simulink model "L1_Control_with_fallback"  (Simulink 7.9)
settings: Solver=ode45  StartTime=0.0  StopTime=300  FixedStep=0.02  MaxStep=0.1  RelTol=1e-3
libraries: simulink x7
settings Model: Creator=prisebor  LastModifiedBy=user
settings SolverCC: ZeroCrossAlgorithm=Adaptive  AutoInsertRateTranBlk=on
settings GRTTargetCC: CombineOutputUpdateFcns=off  GRTInterface=on

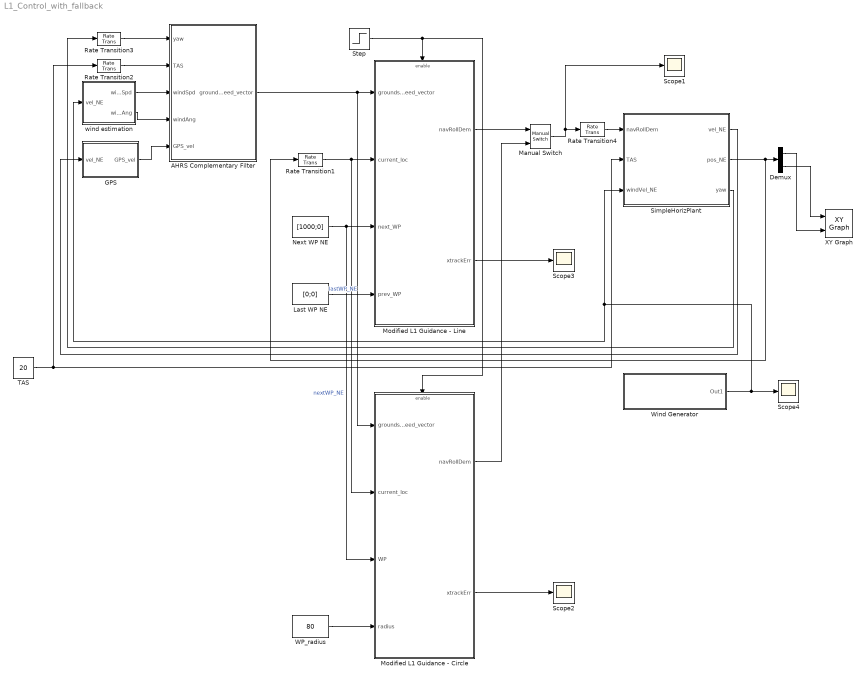
== system L1_Control_with_fallback ==
  AHRS Complementary Filter : Subsystem  TreatAsAtomicUnit=on  SystemSampleTime=0.1
  Demux : Demux  Outputs=2
  GPS : Subsystem  SystemSampleTime=0.2
  Last WP NE : Constant  Value=[0;0]  SampleTime=0.1
  Manual Switch : simulink/Signal Routing/Manual Switch  sw=1  action=0  varsize=off
  Modified L1 Guidance - Circle : Subsystem  TreatAsAtomicUnit=on  SystemSampleTime=0.1  mask{period=20, dampingRatio=0.71, loitDirn=-1}
      mask prompts: period "Tracking Loop Period (sec) - set to 15 times total loop delay"; dampingRatio "Tracking Loop Theoretical Damping Ratio"; loitDirn "Loiter Direction [1 , -1] - 1 for RH, -1 for LH"
  Modified L1 Guidance - Line : Subsystem  TreatAsAtomicUnit=on  SystemSampleTime=0.1  mask{period=20, dampingRatio=0.71, fallbackEnable=1}
      mask prompts: period "Tracking Loop Period (sec) - set to 15 times total loop delay"; dampingRatio "Tracking Loop Theoretical Damping Ratio"; fallbackEnable "Enables fallback mode [1=enabled, 0=disabled]"
  Next WP NE : Constant  Value=[1000;0]  SampleTime=0.1
  Rate Transition1 : RateTransition  OutPortSampleTime=0.1
  Rate Transition2 : RateTransition  OutPortSampleTime=0.1
  Rate Transition3 : RateTransition  OutPortSampleTime=0.1
  Rate Transition4 : RateTransition  OutPortSampleTime=0
  Scope{1..4} (4 alike) : Scope
      Scope2 settings: SaveName=ScopeData2
      Scope4 settings: YMin=-15  SaveName=ScopeData3
  SimpleHorizPlant : Subsystem
  Step : Step  SampleTime=0
  TAS : Constant  Value=20  SampleTime=0
  WP_radius : Constant  Value=80  SampleTime=0.1
  Wind Generator : Subsystem
  XY Graph : simulink/Sinks/XY Graph  xmin=-1000  xmax=1000  ymin=-1000  ymax=1000  st=-1
  wind estimation : Subsystem  SystemSampleTime=0.2
  wires:
  Next WP NE/1 -> Modified L1 Guidance - Circle/3(WP), Modified L1 Guidance - Line/3(next_WP)  "nextWP_NE"
  Last WP NE/1 -> Modified L1 Guidance - Line/4(prev_WP)  "lastWP_NE"
  SimpleHorizPlant/2(pos_NE) -> Rate Transition1/1, Demux/1
  TAS/1 -> SimpleHorizPlant/2(TAS), Rate Transition2/1
  SimpleHorizPlant/3(yaw) -> Rate Transition3/1
  Wind Generator/1(Out1) -> SimpleHorizPlant/3(windVel_NE), wind estimation/1(vel_NE), Scope4/1
  Modified L1 Guidance - Line/1(navRollDem) -> Manual Switch/1
  Rate Transition1/1 -> Modified L1 Guidance - Circle/2(current_loc), Modified L1 Guidance - Line/2(current_loc)
  Rate Transition4/1 -> SimpleHorizPlant/1(navRollDem)
  wind estimation/1(windSpd) -> AHRS Complementary Filter/3(windSpd)
  wind estimation/2(windAng) -> AHRS Complementary Filter/4(windAng)
  Rate Transition3/1 -> AHRS Complementary Filter/1(yaw)
  Rate Transition2/1 -> AHRS Complementary Filter/2(TAS)
  SimpleHorizPlant/1(vel_NE) -> GPS/1(vel_NE)
  GPS/1(GPS_vel) -> AHRS Complementary Filter/5(GPS_vel)
  AHRS Complementary Filter/1(groundspeed_vector) -> Modified L1 Guidance - Circle/1(groundspeed_vector), Modified L1 Guidance - Line/1(groundspeed_vector)
  WP_radius/1 -> Modified L1 Guidance - Circle/4(radius)
  Step/1 -> Modified L1 Guidance - Circle/Enable, Modified L1 Guidance - Line/Enable
  Demux/1 -> XY Graph/2
  Demux/2 -> XY Graph/1
  Manual Switch/1 -> Scope1/1, Rate Transition4/1
  Modified L1 Guidance - Circle/1(navRollDem) -> Manual Switch/2
  Modified L1 Guidance - Circle/2(xtrackErr) -> Scope2/1
  Modified L1 Guidance - Line/2(xtrackErr) -> Scope3/1

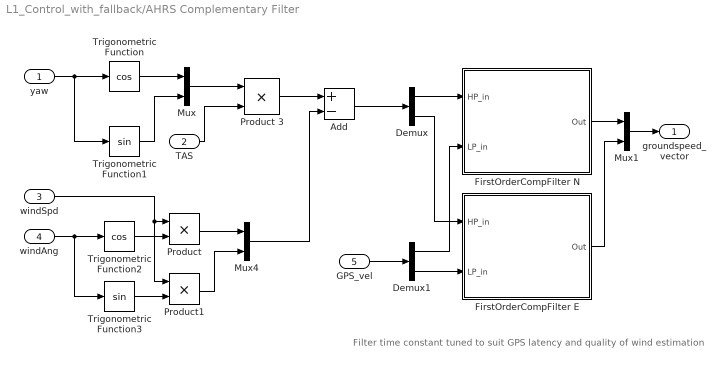
== system L1_Control_with_fallback/AHRS Complementary Filter ==
  note: Filter time constant tuned to suit GPS latency and quality of wind estimation
  yaw : Inport
  TAS : Inport  Port=2
  windSpd : Inport  Port=3
  windAng : Inport  Port=4
  GPS_vel : Inport  Port=5
  Add : Sum  Inputs=+-
  Demux : Demux  Outputs=2
  Demux1 : Demux  Outputs=2
  FirstOrderCompFilter E : Subsystem  mask{beta=0.1}
      mask prompts: beta "Beta=dt/Tau, Tau = filter time constant (sec), dt = filter time step (sec)"
  FirstOrderCompFilter N : Subsystem  mask{beta=0.1}
      mask prompts: beta "Beta=dt/Tau, Tau = filter time constant (sec), dt = filter time step (sec)"
  Mux : Mux  Inputs=2
  Mux1 : Mux  Inputs=2
  Mux4 : Mux  Inputs=2
  Product : Product  RndMeth=Zero
  Product 3 : Product  RndMeth=Zero
  Product1 : Product  RndMeth=Zero
  Trigonometric Function : Trigonometry  Operator=cos
  Trigonometric Function1 : Trigonometry
  Trigonometric Function2 : Trigonometry  Operator=cos
  Trigonometric Function3 : Trigonometry
  groundspeed_vector : Outport
  wires:
  yaw/1 -> Trigonometric Function/1, Trigonometric Function1/1
  Trigonometric Function/1 -> Mux/1
  Trigonometric Function1/1 -> Mux/2
  Mux/1 -> Product 3/1
  Demux/1 -> FirstOrderCompFilter N/1(HP_in)
  Demux1/1 -> FirstOrderCompFilter N/2(LP_in)
  TAS/1 -> Product 3/2
  GPS_vel/1 -> Demux1/1
  Mux1/1 -> groundspeed_vector/1
  FirstOrderCompFilter N/1(Out) -> Mux1/1
  Demux/2 -> FirstOrderCompFilter E/1(HP_in)
  Demux1/2 -> FirstOrderCompFilter E/2(LP_in)
  FirstOrderCompFilter E/1(Out) -> Mux1/2
  Product 3/1 -> Add/1
  Mux4/1 -> Add/2
  Add/1 -> Demux/1
  windAng/1 -> Trigonometric Function2/1, Trigonometric Function3/1
  Trigonometric Function2/1 -> Product/2
  Trigonometric Function3/1 -> Product1/2
  windSpd/1 -> Product/1, Product1/1
  Product/1 -> Mux4/1
  Product1/1 -> Mux4/2

== system L1_Control_with_fallback/GPS ==
  note: UBlox 4Hz output
  note: Cheapo 1Hz output
  vel_NE : Inport
  Integer Delay : Delay  InputProcessing=Inherited
  Integer Delay1 : Delay  DelayLength=8  InputProcessing=Inherited
  Manual Switch : simulink/Signal Routing/Manual Switch  sw=1  action=0  varsize=off
  Rate Transition1 : RateTransition  OutPortSampleTime=0.25
  Rate Transition2 : RateTransition  Deterministic=off  OutPortSampleTime=0.1
  Rate Transition3 : RateTransition  OutPortSampleTime=1
  Rate Transition4 : RateTransition  OutPortSampleTime=0.1
  GPS_vel : Outport
  wires:
  vel_NE/1 -> Rate Transition1/1, Rate Transition3/1
  Rate Transition1/1 -> Rate Transition2/1
  Rate Transition2/1 -> Integer Delay/1
  Rate Transition3/1 -> Rate Transition4/1
  Rate Transition4/1 -> Integer Delay1/1
  Integer Delay1/1 -> Manual Switch/2
  Integer Delay/1 -> Manual Switch/1
  Manual Switch/1 -> GPS_vel/1

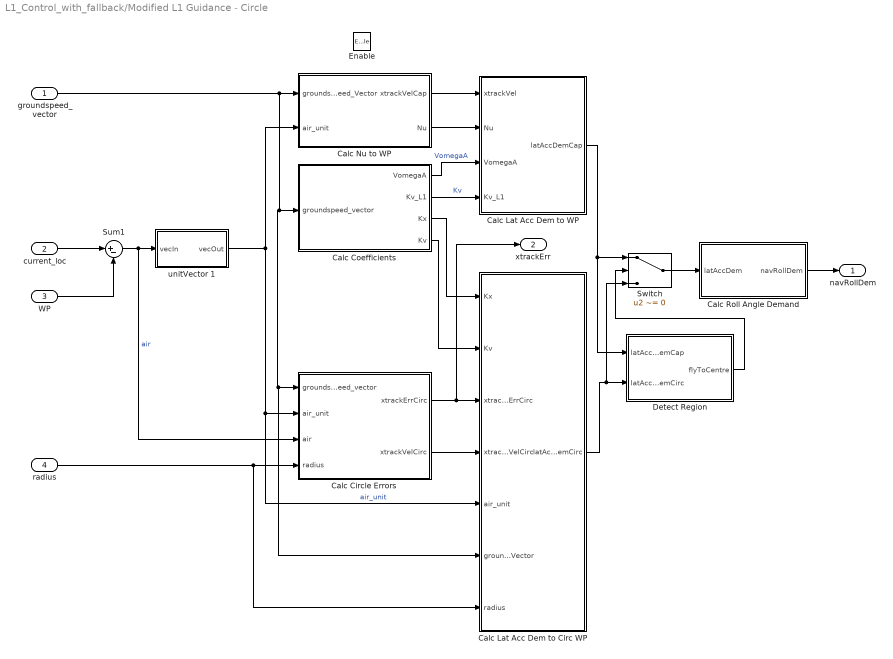
== system L1_Control_with_fallback/Modified L1 Guidance - Circle ==
  groundspeed_vector : Inport
  current_loc : Inport  Port=2
  WP : Inport  Port=3
  radius : Inport  Port=4
  Enable : EnablePort
  Calc Circle Errors : Subsystem
  Calc Coefficients : Subsystem
  Calc Lat Acc Dem to Circ WP : Subsystem
  Calc Lat Acc Dem to WP : Subsystem
  Calc Nu to WP : Subsystem
  Calc Roll Angle Demand : Subsystem
  Detect Region : Subsystem
  Sum1 : Sum  Inputs=|+-
  Switch : Switch  Criteria=u2 ~= 0
  unitVector 1 : Subsystem
  navRollDem : Outport
  xtrackErr : Outport  Port=2
  wires:
  Calc Roll Angle Demand/1(navRollDem) -> navRollDem/1
  groundspeed_vector/1 -> Calc Nu to WP/1(groundspeed_Vector), Calc Lat Acc Dem to Circ WP/6(groundspeed_Vector), Calc Circle Errors/1(groundspeed_vector), Calc Coefficients/1(groundspeed_vector)
  WP/1 -> Sum1/2
  current_loc/1 -> Sum1/1
  Sum1/1 -> Calc Circle Errors/3(air), unitVector 1/1(vecIn)  "air"
  Calc Nu to WP/1(xtrackVelCap) -> Calc Lat Acc Dem to WP/1(xtrackVel)
  Calc Nu to WP/2(Nu) -> Calc Lat Acc Dem to WP/2(Nu)
  Calc Coefficients/1(VomegaA) -> Calc Lat Acc Dem to WP/3(VomegaA)  "VomegaA"
  Calc Coefficients/2(Kv_L1) -> Calc Lat Acc Dem to WP/4(Kv_L1)  "Kv"
  unitVector 1/1(vecOut) -> Calc Lat Acc Dem to Circ WP/5(air_unit), Calc Circle Errors/2(air_unit), Calc Nu to WP/2(air_unit)  "air_unit"
  radius/1 -> Calc Lat Acc Dem to Circ WP/7(radius), Calc Circle Errors/4(radius)
  Calc Circle Errors/2(xtrackVelCirc) -> Calc Lat Acc Dem to Circ WP/4(xtrackVelCirc)
  Calc Circle Errors/1(xtrackErrCirc) -> xtrackErr/1, Calc Lat Acc Dem to Circ WP/3(xtrackErrCirc)
  Calc Coefficients/3(Kx) -> Calc Lat Acc Dem to Circ WP/1(Kx)
  Calc Coefficients/4(Kv) -> Calc Lat Acc Dem to Circ WP/2(Kv)
  Switch/1 -> Calc Roll Angle Demand/1(latAccDem)
  Calc Lat Acc Dem to WP/1(latAccDemCap) -> Detect Region/1(latAccDemCap), Switch/1
  Calc Lat Acc Dem to Circ WP/1(latAccDemCirc) -> Detect Region/2(latAccDemCirc), Switch/3
  Detect Region/1(flyToCentre) -> Switch/2

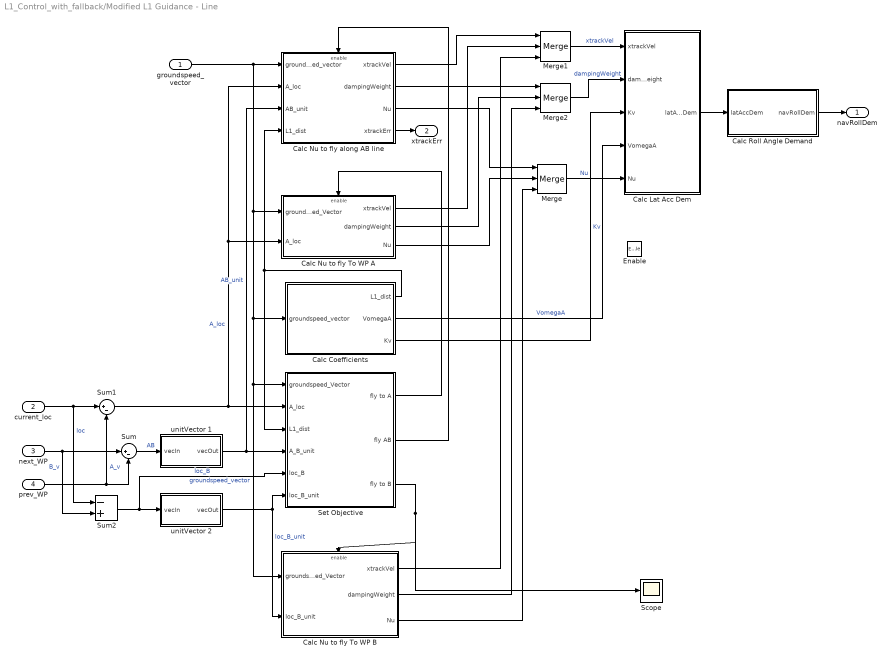
== system L1_Control_with_fallback/Modified L1 Guidance - Line ==
  groundspeed_vector : Inport
  current_loc : Inport  Port=2
  next_WP : Inport  Port=3
  prev_WP : Inport  Port=4
  Enable : EnablePort
  Calc Coefficients : Subsystem
  Calc Lat Acc Dem : Subsystem
  Calc Nu to fly To WP A : Subsystem
  Calc Nu to fly To WP B : Subsystem
  Calc Nu to fly along AB line : Subsystem
  Calc Roll Angle Demand : Subsystem
  Merge : Merge  Inputs=3
  Merge1 : Merge  Inputs=3
  Merge2 : Merge  Inputs=3
  Scope : Scope
      settings: SaveName=ScopeData4
  Set Objective : Subsystem
  Sum : Sum  Inputs=|+-
  Sum1 : Sum  Inputs=|+-
  Sum2 : Sum  Inputs=-+
  unitVector 1 : Subsystem
  unitVector 2 : Subsystem
  navRollDem : Outport
  xtrackErr : Outport  Port=2
  wires:
  Sum1/1 -> Calc Nu to fly along AB line/2(A_loc), Calc Nu to fly To WP A/2(A_loc), Set Objective/2(A_loc)  "A_loc"
  prev_WP/1 -> Sum/2, Sum1/2  "A_v"
  current_loc/1 -> Sum1/1, Sum2/1  "loc"
  next_WP/1 -> Sum/1, Sum2/2  "B_v"
  Calc Coefficients/3(Kv) -> Calc Lat Acc Dem/3(Kv)  "Kv"
  Calc Coefficients/2(VomegaA) -> Calc Lat Acc Dem/4(VomegaA)  "VomegaA"
  Calc Coefficients/1(L1_dist) -> Calc Nu to fly along AB line/4(L1_dist), Set Objective/3(L1_dist)
  groundspeed_vector/1 -> Calc Nu to fly along AB line/1(groundspeed_vector), Calc Nu to fly To WP A/1(groundspeed_Vector), Calc Coefficients/1(groundspeed_vector), Set Objective/1(groundspeed_Vector), Calc Nu to fly To WP B/1(groundspeed_Vector)  "groundspeed_vector"
  Calc Nu to fly along AB line/4(xtrackErr) -> xtrackErr/1
  Sum/1 -> unitVector 1/1(vecIn)  "AB"
  unitVector 1/1(vecOut) -> Calc Nu to fly along AB line/3(AB_unit), Set Objective/4(A_B_unit)  "AB_unit"
  Set Objective/1(fly to A) -> Calc Nu to fly To WP A/Enable
  Merge/1 -> Calc Lat Acc Dem/5(Nu)  "Nu"
  Calc Nu to fly along AB line/3(Nu) -> Merge/1
  Calc Nu to fly To WP A/3(Nu) -> Merge/2
  Merge1/1 -> Calc Lat Acc Dem/1(xtrackVel)  "xtrackVel"
  Calc Nu to fly along AB line/1(xtrackVel) -> Merge1/1
  Calc Nu to fly To WP A/1(xtrackVel) -> Merge1/2
  Calc Nu to fly along AB line/2(dampingWeight) -> Merge2/1
  Merge2/1 -> Calc Lat Acc Dem/2(dampingWeight)  "dampingWeight"
  Calc Nu to fly To WP A/2(dampingWeight) -> Merge2/2
  Calc Lat Acc Dem/1(latAccDem) -> Calc Roll Angle Demand/1(latAccDem)
  Calc Roll Angle Demand/1(navRollDem) -> navRollDem/1
  Set Objective/2(fly AB) -> Calc Nu to fly along AB line/Enable
  Sum2/1 -> unitVector 2/1(vecIn), Set Objective/5(loc_B)  "loc_B"
  unitVector 2/1(vecOut) -> Set Objective/6(loc_B_unit), Calc Nu to fly To WP B/2(loc_B_unit)  "loc_B_unit"
  Set Objective/3(fly to B) -> Calc Nu to fly To WP B/Enable, Scope/1
  Calc Nu to fly To WP B/1(xtrackVel) -> Merge1/3
  Calc Nu to fly To WP B/2(dampingWeight) -> Merge2/3
  Calc Nu to fly To WP B/3(Nu) -> Merge/3

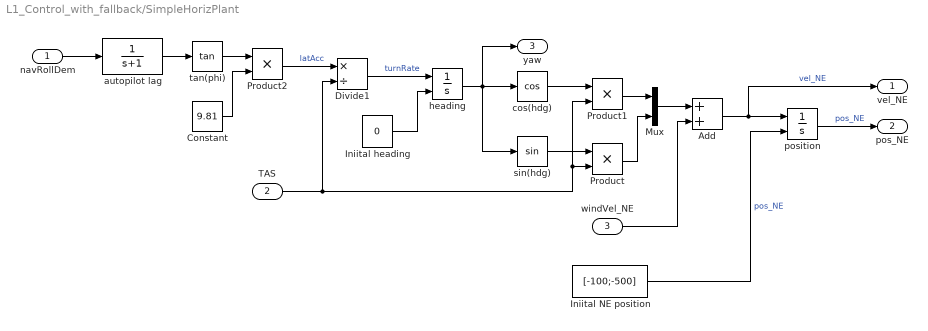
== system L1_Control_with_fallback/SimpleHorizPlant ==
  navRollDem : Inport
  TAS : Inport  Port=2
  windVel_NE : Inport  Port=3
  Add : Sum
  Constant : Constant  Value=9.81
  Divide1 : Product  Inputs=*/
  Iniital NE position : Constant  Value=[-100;-500]
  Iniital heading : Constant  Value=0
  Mux : Mux  Inputs=2
  Product : Product  RndMeth=Zero
  Product1 : Product  RndMeth=Zero
  Product2 : Product  Inputs=**
  autopilot lag : TransferFcn  Denominator=[1.0 1]
  cos(hdg) : Trigonometry  Operator=cos
  heading : Integrator  InitialConditionSource=external  InitialCondition=pi
  position : Integrator  InitialConditionSource=external
  sin(hdg) : Trigonometry
  tan(phi) : Trigonometry  Operator=tan
  vel_NE : Outport
  pos_NE : Outport  Port=2
  yaw : Outport  Port=3
  wires:
  Iniital NE position/1 -> position/2  "pos_NE"
  cos(hdg)/1 -> Product1/1
  TAS/1 -> Product1/2, Product/2, Divide1/2
  windVel_NE/1 -> Add/2
  heading/1 -> sin(hdg)/1, yaw/1, cos(hdg)/1
  sin(hdg)/1 -> Product/1
  position/1 -> pos_NE/1  "pos_NE"
  Mux/1 -> Add/1
  Product/1 -> Mux/2
  Product1/1 -> Mux/1
  Add/1 -> vel_NE/1, position/1  "vel_NE"
  autopilot lag/1 -> tan(phi)/1
  navRollDem/1 -> autopilot lag/1
  Iniital heading/1 -> heading/2
  tan(phi)/1 -> Product2/1
  Product2/1 -> Divide1/1  "latAcc"
  Divide1/1 -> heading/1  "turnRate"
  Constant/1 -> Product2/2

== system L1_Control_with_fallback/Wind Generator ==
  Add : Sum
  Band-Limited White Noise : simulink/Sources/Band-Limited White Noise  Cov=[0.1]  Ts=0.1  seed=[23341]
  Band-Limited White Noise1 : simulink/Sources/Band-Limited White Noise  Cov=[0.1]  Ts=0.1  seed=[23342]
  Gain : Gain  Gain=25
  Gain1 : Gain  Gain=25
  Mux : Mux  Inputs=2
  Transfer Fcn : TransferFcn  Denominator=[10 1]
  Transfer Fcn1 : TransferFcn  Denominator=[10 1]
  windVelNE : Constant  Value=[0;-20]
  Out1 : Outport
  wires:
  Band-Limited White Noise/1 -> Gain/1
  Band-Limited White Noise1/1 -> Gain1/1
  Gain/1 -> Transfer Fcn/1
  Gain1/1 -> Transfer Fcn1/1
  Transfer Fcn1/1 -> Mux/2
  windVelNE/1 -> Add/2
  Add/1 -> Out1/1
  Transfer Fcn/1 -> Mux/1
  Mux/1 -> Add/1

== system L1_Control_with_fallback/wind estimation ==
  note: angle wind is coming from - hence sign change
  vel_NE : Inport
  Demux : Demux  Outputs=2
  Dot Product : DotProduct  InputSameDT=on  OutDataTypeStr=Inherit: Inherit via internal rule
  Gain : Gain  Gain=-1
  Rate Transition2 : RateTransition  OutPortSampleTime=0.1
  Rate Transition5 : RateTransition  OutPortSampleTime=0.1
  Sqrt : Sqrt  SaturateOnIntegerOverflow=on
  Sum : Sum  Inputs=|++
  Sum1 : Sum  Inputs=|++
  Trigonometric Function : Trigonometry  Operator=atan2
  wind angle error : Constant  Value=0.1
  wind speed error : Constant  Value=-1
  windSpd : Outport
  windAng : Outport  Port=2
  wires:
  vel_NE/1 -> Rate Transition5/1
  Rate Transition2/1 -> Demux/1, Dot Product/1, Dot Product/2
  Demux/2 -> Trigonometric Function/1
  Demux/1 -> Trigonometric Function/2
  Trigonometric Function/1 -> Gain/1
  Dot Product/1 -> Sqrt/1
  Rate Transition5/1 -> Rate Transition2/1
  Gain/1 -> Sum/1
  Sum/1 -> windAng/1
  Sqrt/1 -> Sum1/1
  Sum1/1 -> windSpd/1
  wind angle error/1 -> Sum/2
  wind speed error/1 -> Sum1/2

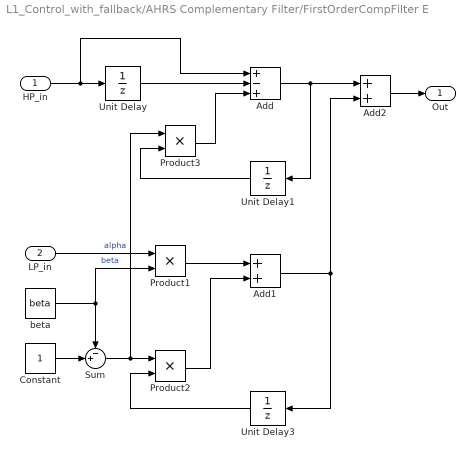
== system L1_Control_with_fallback/AHRS Complementary Filter/FirstOrderCompFilter E ==
  HP_in : Inport
  LP_in : Inport  Port=2
  Add : Sum  Inputs=+-+
  Add1 : Sum
  Add2 : Sum
  Constant : Constant
  Product1 : Product  RndMeth=Zero
  Product2 : Product  RndMeth=Zero
  Product3 : Product  RndMeth=Zero
  Sum : Sum  Inputs=-+|
  Unit Delay : UnitDelay  SampleTime=-1
  Unit Delay1 : UnitDelay  SampleTime=-1
  Unit Delay3 : UnitDelay  SampleTime=-1
  beta : Constant  Value=beta
  Out : Outport
  wires:
  Constant/1 -> Sum/2
  Unit Delay1/1 -> Product3/2
  Product3/1 -> Add/3
  Product2/1 -> Add1/2
  Unit Delay3/1 -> Product2/2
  Sum/1 -> Product3/1, Product2/1  "alpha"
  beta/1 -> Sum/1, Product1/2  "beta"
  Add2/1 -> Out/1
  LP_in/1 -> Product1/1
  HP_in/1 -> Add/1, Unit Delay/1
  Product1/1 -> Add1/1
  Add1/1 -> Add2/2, Unit Delay3/1
  Add/1 -> Add2/1, Unit Delay1/1
  Unit Delay/1 -> Add/2

== system L1_Control_with_fallback/AHRS Complementary Filter/FirstOrderCompFilter N ==
  HP_in : Inport
  LP_in : Inport  Port=2
  Add : Sum  Inputs=+-+
  Add1 : Sum
  Add2 : Sum
  Constant : Constant
  Product1 : Product  RndMeth=Zero
  Product2 : Product  RndMeth=Zero
  Product3 : Product  RndMeth=Zero
  Sum : Sum  Inputs=-+|
  Unit Delay : UnitDelay  SampleTime=-1
  Unit Delay1 : UnitDelay  SampleTime=-1
  Unit Delay3 : UnitDelay  SampleTime=-1
  beta : Constant  Value=beta
  Out : Outport
  wires:
  Unit Delay/1 -> Add/2
  Add/1 -> Unit Delay1/1, Add2/1
  Add1/1 -> Unit Delay3/1, Add2/2
  Product1/1 -> Add1/1
  HP_in/1 -> Unit Delay/1, Add/1
  LP_in/1 -> Product1/1
  Add2/1 -> Out/1
  beta/1 -> Product1/2, Sum/1  "beta"
  Sum/1 -> Product2/1, Product3/1  "alpha"
  Unit Delay3/1 -> Product2/2
  Product2/1 -> Add1/2
  Product3/1 -> Add/3
  Unit Delay1/1 -> Product3/2
  Constant/1 -> Sum/2

== system L1_Control_with_fallback/Modified L1 Guidance - Circle/Calc Circle Errors ==
  groundspeed_vector : Inport
  air_unit : Inport  Port=2
  air : Inport  Port=3
  radius : Inport  Port=4
  Add 2 : Sum  Inputs=+-
  Dot Product : DotProduct  InputSameDT=on  OutDataTypeStr=Inherit: Inherit via internal rule
  Dot Product1 : DotProduct  InputSameDT=on  OutDataTypeStr=Inherit: Inherit via internal rule
  Sqrt : Sqrt  SaturateOnIntegerOverflow=on
  xtrackErrCirc : Outport
  xtrackVelCirc : Outport  Port=2
  wires:
  air_unit/1 -> Dot Product/2
  groundspeed_vector/1 -> Dot Product/1  "groundspeed_vector"
  air/1 -> Dot Product1/2, Dot Product1/1
  Dot Product1/1 -> Sqrt/1
  Sqrt/1 -> Add 2/1
  radius/1 -> Add 2/2
  Dot Product/1 -> xtrackVelCirc/1
  Add 2/1 -> xtrackErrCirc/1

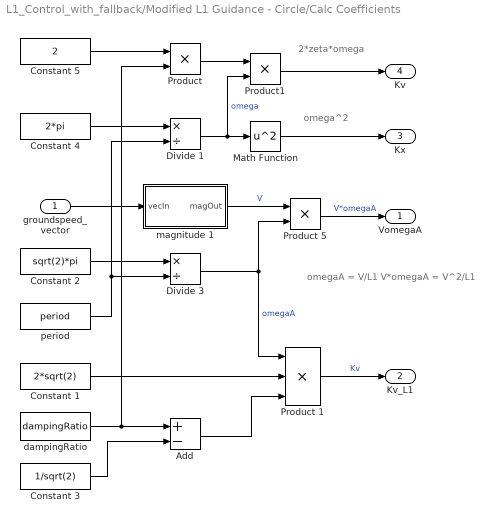
== system L1_Control_with_fallback/Modified L1 Guidance - Circle/Calc Coefficients ==
  note: omega^2
  note: 2*zeta*omega
  note: omegaA = V/L1
      | V*omegaA = V^2/L1
  groundspeed_vector : Inport
  Add : Sum  Inputs=+-
  Constant 1 : Constant  Value=2*sqrt(2)
  Constant 2 : Constant  Value=sqrt(2)*pi
  Constant 3 : Constant  Value=1/sqrt(2)
  Constant 4 : Constant  Value=2*pi
  Constant 5 : Constant  Value=2
  Divide 1 : Product  Inputs=*/
  Divide 3 : Product  Inputs=*/
  Math Function : Math  Operator=square  SaturateOnIntegerOverflow=on
  Product : Product  Inputs=**
  Product 1 : Product  Inputs=3  RndMeth=Zero
  Product 5 : Product  RndMeth=Zero
  Product1 : Product  Inputs=**
  dampingRatio : Constant  Value=dampingRatio
  magnitude 1 : Subsystem
  period : Constant  Value=period
  VomegaA : Outport
  Kv_L1 : Outport  Port=2
  Kx : Outport  Port=3
  Kv : Outport  Port=4
  wires:
  Product 1/1 -> Kv_L1/1  "Kv"
  Product 5/1 -> VomegaA/1  "V*omegaA"
  groundspeed_vector/1 -> magnitude 1/1(vecIn)
  Constant 1/1 -> Product 1/2
  Add/1 -> Product 1/3
  magnitude 1/1(magOut) -> Product 5/1  "V"
  Divide 3/1 -> Product 1/1, Product 5/2  "omegaA"
  Constant 3/1 -> Add/2
  dampingRatio/1 -> Product/2, Add/1
  period/1 -> Divide 1/2, Divide 3/2
  Constant 2/1 -> Divide 3/1
  Constant 4/1 -> Divide 1/1
  Divide 1/1 -> Product1/2, Math Function/1  "omega"
  Math Function/1 -> Kx/1
  Constant 5/1 -> Product/1
  Product/1 -> Product1/1
  Product1/1 -> Kv/1

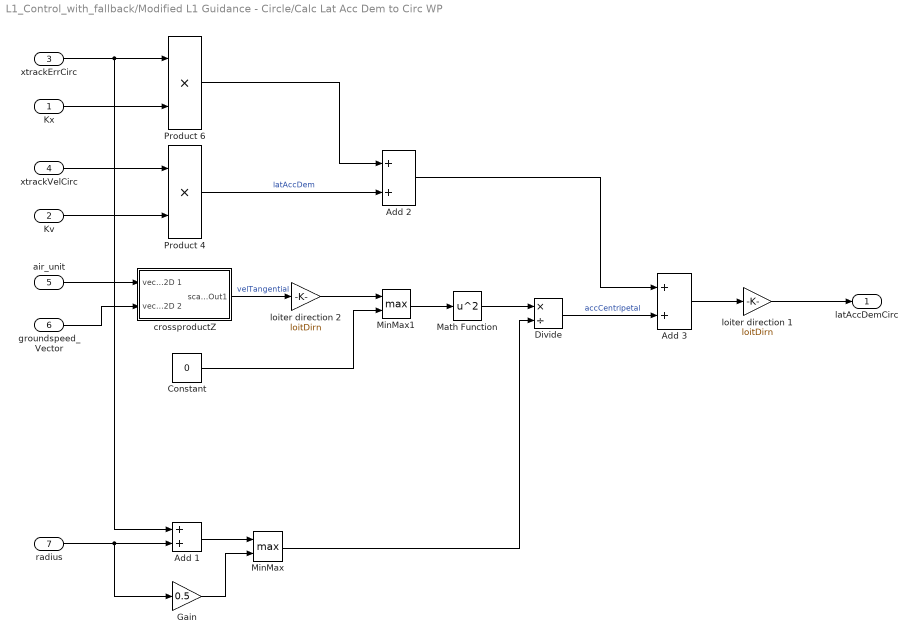
== system L1_Control_with_fallback/Modified L1 Guidance - Circle/Calc Lat Acc Dem to Circ WP ==
  Kx : Inport
  Kv : Inport  Port=2
  xtrackErrCirc : Inport  Port=3
  xtrackVelCirc : Inport  Port=4
  air_unit : Inport  Port=5
  groundspeed_Vector : Inport  Port=6
  radius : Inport  Port=7
  Add 1 : Sum
  Add 2 : Sum  Inputs=2
  Add 3 : Sum  Inputs=2
  Constant : Constant  Value=0
  Divide : Product  Inputs=*/
  Gain : Gain  Gain=0.5
  Math Function : Math  Operator=square  SaturateOnIntegerOverflow=on
  MinMax : MinMax  Function=max  Inputs=2
  MinMax1 : MinMax  Function=max  Inputs=2
  Product 4 : Product  RndMeth=Zero
  Product 6 : Product  RndMeth=Zero
  crossproductZ : Subsystem
  loiter direction 1 : Gain  Gain=loitDirn
  loiter direction 2 : Gain  Gain=loitDirn
  latAccDemCirc : Outport
  wires:
  Kv/1 -> Product 4/2
  xtrackVelCirc/1 -> Product 4/1
  Product 4/1 -> Add 2/2  "latAccDem"
  Product 6/1 -> Add 2/1
  xtrackErrCirc/1 -> Add 1/1, Product 6/1
  Kx/1 -> Product 6/2
  air_unit/1 -> crossproductZ/1(vecIn2D 1)
  groundspeed_Vector/1 -> crossproductZ/2(vecIn2D 2)
  Add 1/1 -> MinMax/1
  crossproductZ/1(scalarOut1) -> loiter direction 2/1  "velTangential"
  Math Function/1 -> Divide/1
  MinMax/1 -> Divide/2
  radius/1 -> Gain/1, Add 1/2
  Gain/1 -> MinMax/2
  MinMax1/1 -> Math Function/1
  Constant/1 -> MinMax1/2
  Add 3/1 -> loiter direction 1/1
  Add 2/1 -> Add 3/1
  Divide/1 -> Add 3/2  "accCentripetal"
  loiter direction 2/1 -> MinMax1/1
  loiter direction 1/1 -> latAccDemCirc/1

== system L1_Control_with_fallback/Modified L1 Guidance - Circle/Calc Lat Acc Dem to WP ==
  note: additional damping
  xtrackVel : Inport
  Nu : Inport  Port=2
  VomegaA : Inport  Port=3
  Kv_L1 : Inport  Port=4
  Add 2 : Sum
  "Constant 2 " : Constant  Value=2
  Product 4 : Product  RndMeth=Zero
  Product 6 : Product  RndMeth=Zero
  Product 7 : Product  RndMeth=Zero
  sin(Nu) : Trigonometry
  latAccDemCap : Outport
  wires:
  Nu/1 -> sin(Nu)/1
  VomegaA/1 -> Product 7/2
  Product 7/1 -> latAccDemCap/1
  Kv_L1/1 -> Product 6/2
  xtrackVel/1 -> Product 6/1
  Add 2/1 -> Product 7/1
  Product 6/1 -> Add 2/1
  Product 4/1 -> Add 2/2  "latAccDem"
  "Constant 2 "/1 -> Product 4/1
  sin(Nu)/1 -> Product 4/2

== system L1_Control_with_fallback/Modified L1 Guidance - Circle/Calc Nu to WP ==
  groundspeed_Vector : Inport
  air_unit : Inport  Port=2
  Dot Product : DotProduct  InputSameDT=on  OutDataTypeStr=Inherit: Inherit via internal rule
  Gain : Gain  Gain=-1
  Saturation : Saturate  UpperLimit=pi/2  LowerLimit=-pi/2
  atan2 : Trigonometry  Operator=atan2
  crossproductZ : Subsystem
  xtrackVelCap : Outport
  Nu : Outport  Port=2
  wires:
  atan2/1 -> Saturation/1  "Nu"
  groundspeed_Vector/1 -> Dot Product/1, crossproductZ/2(vecIn2D 2)
  Dot Product/1 -> Gain/1  "ltrackVelCap"
  crossproductZ/1(scalarOut1) -> atan2/1, xtrackVelCap/1  "xtrackVelCap"
  air_unit/1 -> Dot Product/2, crossproductZ/1(vecIn2D 1)
  Gain/1 -> atan2/2
  Saturation/1 -> Nu/1

== system L1_Control_with_fallback/Modified L1 Guidance - Circle/Calc Roll Angle Demand ==
  latAccDem : Inport
  Divide 2 : Product  Inputs=*/
  Saturation1 : Saturate  UpperLimit=pi/4  LowerLimit=-pi/4
  atan : Trigonometry  Operator=atan
  gravity : Constant  Value=9.8
  navRollDem : Outport
  wires:
  Saturation1/1 -> navRollDem/1
  latAccDem/1 -> Divide 2/1
  gravity/1 -> Divide 2/2
  Divide 2/1 -> atan/1
  atan/1 -> Saturation1/1

== system L1_Control_with_fallback/Modified L1 Guidance - Circle/Detect Region ==
  latAccDemCap : Inport
  latAccDemCirc : Inport  Port=2
  Compare To Zero : simulink/Logic and Bit Operations/Compare To Zero  relop=>  OutDataTypeStr=uint8
  Logical Operator : Logic  AllPortsSameDT=off  OutDataTypeStr=boolean
  Logical Operator1 : Logic  Operator=OR  AllPortsSameDT=off  OutDataTypeStr=boolean
  Logical Operator2 : Logic  Operator=NOT  AllPortsSameDT=off  OutDataTypeStr=boolean
  Logical Operator3 : Logic  AllPortsSameDT=off  OutDataTypeStr=boolean
  Loiter Direction : Constant  Value=loitDirn
  Relational Operator 2 : RelationalOperator  Operator=<  OutDataTypeStr=boolean
  Relational Operator1 : RelationalOperator  Operator=>  OutDataTypeStr=boolean
  flyToCentre : Outport
  wires:
  latAccDemCap/1 -> Relational Operator 2/1, Relational Operator1/1
  latAccDemCirc/1 -> Relational Operator 2/2, Relational Operator1/2
  Loiter Direction/1 -> Compare To Zero/1
  Relational Operator 2/1 -> Logical Operator/1
  Compare To Zero/1 -> Logical Operator2/1, Logical Operator/2
  Logical Operator/1 -> Logical Operator1/1
  Logical Operator1/1 -> flyToCentre/1
  Relational Operator1/1 -> Logical Operator3/2
  Logical Operator2/1 -> Logical Operator3/1
  Logical Operator3/1 -> Logical Operator1/2

== system L1_Control_with_fallback/Modified L1 Guidance - Circle/unitVector 1 ==
  vecIn : Inport
  Divide : Product  Inputs=*/
  Dot Product : DotProduct  InputSameDT=on  OutDataTypeStr=Inherit: Inherit via internal rule
  Sqrt : Sqrt  SaturateOnIntegerOverflow=on
  vecOut : Outport
  wires:
  vecIn/1 -> Divide/1, Dot Product/2, Dot Product/1
  Sqrt/1 -> Divide/2
  Dot Product/1 -> Sqrt/1
  Divide/1 -> vecOut/1

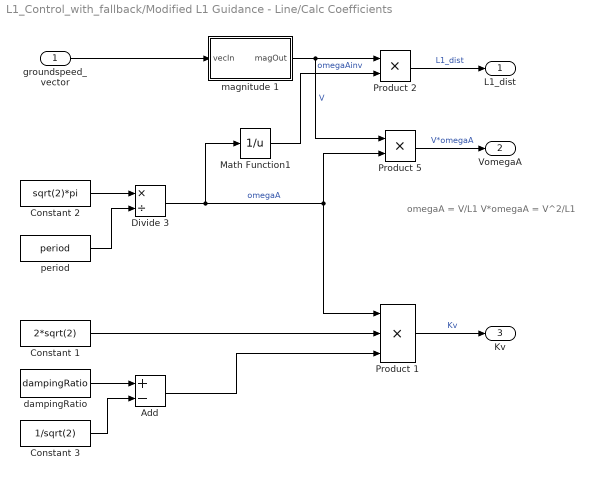
== system L1_Control_with_fallback/Modified L1 Guidance - Line/Calc Coefficients ==
  note: omegaA = V/L1
      | V*omegaA = V^2/L1
  groundspeed_vector : Inport
  Add : Sum  Inputs=+-
  Constant 1 : Constant  Value=2*sqrt(2)
  Constant 2 : Constant  Value=sqrt(2)*pi
  Constant 3 : Constant  Value=1/sqrt(2)
  Divide 3 : Product  Inputs=*/
  Math Function1 : Math  Operator=reciprocal  SaturateOnIntegerOverflow=on
  Product 1 : Product  Inputs=3  RndMeth=Zero
  Product 2 : Product  RndMeth=Zero
  Product 5 : Product  RndMeth=Zero
  dampingRatio : Constant  Value=dampingRatio
  magnitude 1 : Subsystem
  period : Constant  Value=period
  L1_dist : Outport
  VomegaA : Outport  Port=2
  Kv : Outport  Port=3
  wires:
  Constant 2/1 -> Divide 3/1
  period/1 -> Divide 3/2
  dampingRatio/1 -> Add/1
  Constant 3/1 -> Add/2
  Divide 3/1 -> Math Function1/1, Product 1/1, Product 5/2  "omegaA"
  magnitude 1/1(magOut) -> Product 5/1, Product 2/1  "V"
  Add/1 -> Product 1/3
  Constant 1/1 -> Product 1/2
  Math Function1/1 -> Product 2/2  "omegaAinv"
  groundspeed_vector/1 -> magnitude 1/1(vecIn)
  Product 2/1 -> L1_dist/1  "L1_dist"
  Product 5/1 -> VomegaA/1  "V*omegaA"
  Product 1/1 -> Kv/1  "Kv"

== system L1_Control_with_fallback/Modified L1 Guidance - Line/Calc Lat Acc Dem ==
  note: additional damping
  xtrackVel : Inport
  dampingWeight : Inport  Port=2
  Kv : Inport  Port=3
  VomegaA : Inport  Port=4
  Nu : Inport  Port=5
  Add 2 : Sum
  "Constant 2 " : Constant  Value=2
  Product 4 : Product  RndMeth=Zero
  Product 6 : Product  Inputs=3  RndMeth=Zero
  Product 7 : Product  RndMeth=Zero
  sin(Nu) : Trigonometry
  latAccDem : Outport
  wires:
  sin(Nu)/1 -> Product 4/2
  "Constant 2 "/1 -> Product 4/1
  Product 4/1 -> Add 2/2  "latAccDem"
  Product 6/1 -> Add 2/1
  Add 2/1 -> Product 7/1
  xtrackVel/1 -> Product 6/1
  dampingWeight/1 -> Product 6/2
  Kv/1 -> Product 6/3
  Product 7/1 -> latAccDem/1  "latAccDem"
  VomegaA/1 -> Product 7/2
  Nu/1 -> sin(Nu)/1

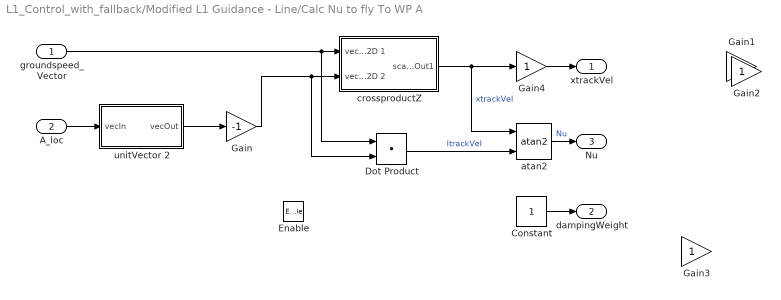
== system L1_Control_with_fallback/Modified L1 Guidance - Line/Calc Nu to fly To WP A ==
  groundspeed_Vector : Inport
  A_loc : Inport  Port=2
  Enable : EnablePort
  Constant : Constant
  Dot Product : DotProduct  InputSameDT=on  OutDataTypeStr=Inherit: Inherit via internal rule
  Gain : Gain  Gain=-1
  Gain{1..4} (4 alike) : Gain
  atan2 : Trigonometry  Operator=atan2
  crossproductZ : Subsystem
  unitVector 2 : Subsystem
  xtrackVel : Outport
  dampingWeight : Outport  Port=2
  Nu : Outport  Port=3
  wires:
  unitVector 2/1(vecOut) -> Gain/1
  Gain/1 -> crossproductZ/2(vecIn2D 2), Dot Product/2
  crossproductZ/1(scalarOut1) -> atan2/1, Gain4/1  "xtrackVel"
  Dot Product/1 -> atan2/2  "ltrackVel"
  groundspeed_Vector/1 -> crossproductZ/1(vecIn2D 1), Dot Product/1
  A_loc/1 -> unitVector 2/1(vecIn)
  atan2/1 -> Nu/1  "Nu"
  Gain4/1 -> xtrackVel/1
  Constant/1 -> dampingWeight/1

== system L1_Control_with_fallback/Modified L1 Guidance - Line/Calc Nu to fly To WP B ==
  groundspeed_Vector : Inport
  loc_B_unit : Inport  Port=2
  Enable : EnablePort
  Constant : Constant
  Dot Product : DotProduct  InputSameDT=on  OutDataTypeStr=Inherit: Inherit via internal rule
  Gain4 : Gain
  atan2 : Trigonometry  Operator=atan2
  crossproductZ : Subsystem
  xtrackVel : Outport
  dampingWeight : Outport  Port=2
  Nu : Outport  Port=3
  wires:
  Constant/1 -> dampingWeight/1
  Gain4/1 -> xtrackVel/1
  atan2/1 -> Nu/1  "Nu"
  groundspeed_Vector/1 -> Dot Product/1, crossproductZ/1(vecIn2D 1)
  Dot Product/1 -> atan2/2  "ltrackVel"
  crossproductZ/1(scalarOut1) -> Gain4/1, atan2/1  "xtrackVel"
  loc_B_unit/1 -> Dot Product/2, crossproductZ/2(vecIn2D 2)

== system L1_Control_with_fallback/Modified L1 Guidance - Line/Calc Nu to fly along AB line ==
  groundspeed_vector : Inport
  A_loc : Inport  Port=2
  AB_unit : Inport  Port=3
  L1_dist : Inport  Port=4
  Enable : EnablePort
  Add 1 : Sum
  Calculate Nu1 Angle : Subsystem
  Calculate Nu2 Angle : Subsystem
  xtrackVel : Outport
  dampingWeight : Outport  Port=2
  Nu : Outport  Port=3
  xtrackErr : Outport  Port=4
  wires:
  Calculate Nu1 Angle/1(Nu1) -> Add 1/2  "Nu1"
  Calculate Nu2 Angle/2(Nu2) -> Add 1/1  "Nu2"
  Calculate Nu1 Angle/3(xtrackErr) -> xtrackErr/1  "xtrackErr"
  groundspeed_vector/1 -> Calculate Nu2 Angle/1(groundspeed_vector)  "groundspeed_vector"
  A_loc/1 -> Calculate Nu1 Angle/1(A_loc)
  L1_dist/1 -> Calculate Nu1 Angle/3(L1_dist)
  Calculate Nu2 Angle/1(xtrackVel) -> xtrackVel/1  "xtrackVel"
  Add 1/1 -> Nu/1  "Nu"
  Calculate Nu1 Angle/2(dampingWeight) -> dampingWeight/1  "dampingWeight"
  AB_unit/1 -> Calculate Nu1 Angle/2(AB_unit), Calculate Nu2 Angle/2(trackUnitVec)  "AB_unit"

== system L1_Control_with_fallback/Modified L1 Guidance - Line/Calc Roll Angle Demand ==
  latAccDem : Inport
  Divide 2 : Product  Inputs=*/
  Saturation1 : Saturate  UpperLimit=pi/4  LowerLimit=-pi/4
  atan : Trigonometry  Operator=atan
  gravity : Constant  Value=9.8
  navRollDem : Outport
  wires:
  atan/1 -> Saturation1/1
  Divide 2/1 -> atan/1
  gravity/1 -> Divide 2/2
  latAccDem/1 -> Divide 2/1
  Saturation1/1 -> navRollDem/1

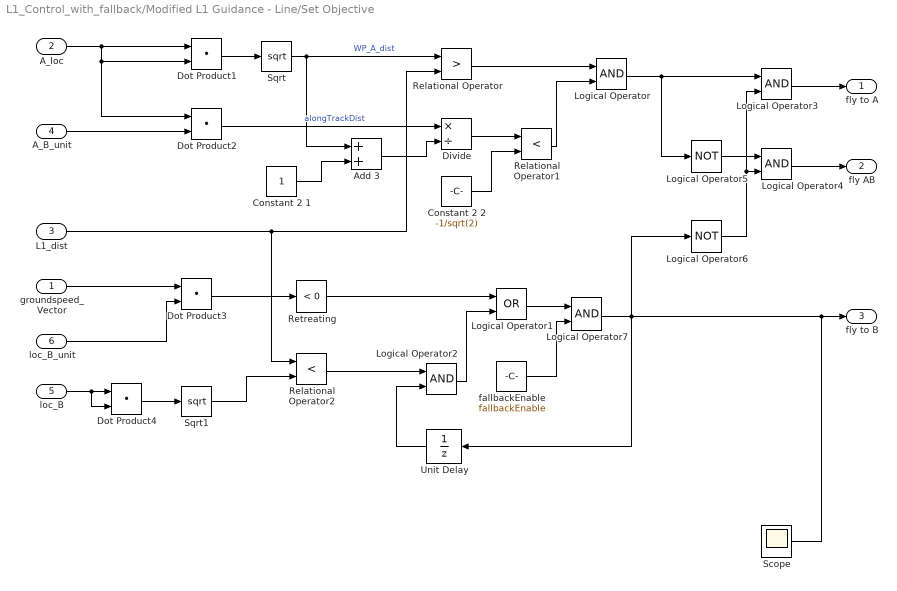
== system L1_Control_with_fallback/Modified L1 Guidance - Line/Set Objective ==
  groundspeed_Vector : Inport
  A_loc : Inport  Port=2
  L1_dist : Inport  Port=3
  A_B_unit : Inport  Port=4
  loc_B : Inport  Port=5
  loc_B_unit : Inport  Port=6
  Add 3 : Sum
  Constant 2 1 : Constant
  Constant 2 2 : Constant  Value=-1/sqrt(2)
  Divide : Product  Inputs=*/
  Dot Product{1..4} (4 alike) : DotProduct  InputSameDT=on  OutDataTypeStr=Inherit: Inherit via internal rule
  Logical Operator{,2..4,7} (5 alike) : Logic  AllPortsSameDT=off  OutDataTypeStr=boolean
  Logical Operator1 : Logic  Operator=OR  AllPortsSameDT=off  OutDataTypeStr=boolean
  Logical Operator5 : Logic  Operator=NOT  AllPortsSameDT=off  OutDataTypeStr=boolean
  Logical Operator6 : Logic  Operator=NOT  AllPortsSameDT=off  OutDataTypeStr=boolean
  Relational Operator : RelationalOperator  Operator=>  OutDataTypeStr=boolean
  Relational Operator1 : RelationalOperator  Operator=<  OutDataTypeStr=boolean
  Relational Operator2 : RelationalOperator  Operator=<  OutDataTypeStr=boolean
  Retreating : simulink/Logic and Bit Operations/Compare To Zero  relop=<  OutDataTypeStr=uint8
  Scope : Scope
      settings: SaveName=ScopeData5
  Sqrt : Sqrt  SaturateOnIntegerOverflow=on
  Sqrt1 : Sqrt  SaturateOnIntegerOverflow=on
  Unit Delay : UnitDelay  SampleTime=-1
  fallbackEnable : Constant  Value=fallbackEnable
  fly to A : Outport
  fly AB : Outport  Port=2
  fly to B : Outport  Port=3
  wires:
  Dot Product1/1 -> Sqrt/1
  Sqrt/1 -> Relational Operator/1, Add 3/1  "WP_A_dist"
  Dot Product2/1 -> Divide/1  "alongTrackDist"
  Add 3/1 -> Divide/2
  Constant 2 1/1 -> Add 3/2
  Divide/1 -> Relational Operator1/1
  Constant 2 2/1 -> Relational Operator1/2
  Relational Operator/1 -> Logical Operator/1
  Relational Operator1/1 -> Logical Operator/2
  A_loc/1 -> Dot Product2/1, Dot Product1/2, Dot Product1/1
  L1_dist/1 -> Relational Operator/2, Relational Operator2/1
  A_B_unit/1 -> Dot Product2/2
  loc_B_unit/1 -> Dot Product3/2
  Dot Product3/1 -> Retreating/1
  Retreating/1 -> Logical Operator1/1
  Logical Operator2/1 -> Logical Operator1/2
  Relational Operator2/1 -> Logical Operator2/1
  Logical Operator1/1 -> Logical Operator7/1
  Unit Delay/1 -> Logical Operator2/2
  Logical Operator/1 -> Logical Operator3/1, Logical Operator5/1
  Logical Operator4/1 -> fly AB/1
  Logical Operator5/1 -> Logical Operator4/1
  Logical Operator6/1 -> Logical Operator4/2, Logical Operator3/2
  Logical Operator3/1 -> fly to A/1
  groundspeed_Vector/1 -> Dot Product3/1
  Dot Product4/1 -> Sqrt1/1
  loc_B/1 -> Dot Product4/1, Dot Product4/2
  Sqrt1/1 -> Relational Operator2/2
  Logical Operator7/1 -> Unit Delay/1, Logical Operator6/1, fly to B/1, Scope/1
  fallbackEnable/1 -> Logical Operator7/2

== system L1_Control_with_fallback/Modified L1 Guidance - Line/unitVector 1 ==
  vecIn : Inport
  Divide : Product  Inputs=*/
  Dot Product : DotProduct  InputSameDT=on  OutDataTypeStr=Inherit: Inherit via internal rule
  Sqrt : Sqrt  SaturateOnIntegerOverflow=on
  vecOut : Outport
  wires:
  Divide/1 -> vecOut/1
  Dot Product/1 -> Sqrt/1
  Sqrt/1 -> Divide/2
  vecIn/1 -> Dot Product/1, Dot Product/2, Divide/1

== system L1_Control_with_fallback/Modified L1 Guidance - Line/unitVector 2 ==
  vecIn : Inport
  Divide : Product  Inputs=*/
  Dot Product : DotProduct  InputSameDT=on  OutDataTypeStr=Inherit: Inherit via internal rule
  Sqrt : Sqrt  SaturateOnIntegerOverflow=on
  vecOut : Outport
  wires:
  vecIn/1 -> Divide/1, Dot Product/2, Dot Product/1
  Sqrt/1 -> Divide/2
  Dot Product/1 -> Sqrt/1
  Divide/1 -> vecOut/1

== system L1_Control_with_fallback/Modified L1 Guidance - Circle/Calc Coefficients/magnitude 1 ==
  vecIn : Inport
  Dot Product : DotProduct  InputSameDT=on  OutDataTypeStr=Inherit: Inherit via internal rule
  Sqrt : Sqrt  SaturateOnIntegerOverflow=on
  magOut : Outport
  wires:
  Sqrt/1 -> magOut/1
  Dot Product/1 -> Sqrt/1
  vecIn/1 -> Dot Product/1, Dot Product/2

== system L1_Control_with_fallback/Modified L1 Guidance - Circle/Calc Lat Acc Dem to Circ WP/crossproductZ ==
  vecIn2D 1 : Inport
  vecIn2D 2 : Inport  Port=2
  Demux : Demux  Outputs=2
  Demux1 : Demux  Outputs=2
  Product : Product  RndMeth=Zero
  Product1 : Product  RndMeth=Zero
  Sum2 : Sum  Inputs=|+-
  scalarOut1 : Outport
  wires:
  Product1/1 -> Sum2/2
  vecIn2D 2/1 -> Demux1/1
  Demux/1 -> Product/1
  Demux/2 -> Product1/1
  vecIn2D 1/1 -> Demux/1
  Demux1/1 -> Product1/2
  Demux1/2 -> Product/2
  Sum2/1 -> scalarOut1/1
  Product/1 -> Sum2/1

== system L1_Control_with_fallback/Modified L1 Guidance - Circle/Calc Nu to WP/crossproductZ ==
  vecIn2D 1 : Inport
  vecIn2D 2 : Inport  Port=2
  Demux : Demux  Outputs=2
  Demux1 : Demux  Outputs=2
  Product : Product  RndMeth=Zero
  Product1 : Product  RndMeth=Zero
  Sum2 : Sum  Inputs=|+-
  scalarOut1 : Outport
  wires:
  Product1/1 -> Sum2/2
  vecIn2D 2/1 -> Demux1/1
  Demux/1 -> Product/1
  Demux/2 -> Product1/1
  vecIn2D 1/1 -> Demux/1
  Demux1/1 -> Product1/2
  Demux1/2 -> Product/2
  Sum2/1 -> scalarOut1/1
  Product/1 -> Sum2/1

== system L1_Control_with_fallback/Modified L1 Guidance - Line/Calc Coefficients/magnitude 1 ==
  vecIn : Inport
  Dot Product : DotProduct  InputSameDT=on  OutDataTypeStr=Inherit: Inherit via internal rule
  Sqrt : Sqrt  SaturateOnIntegerOverflow=on
  magOut : Outport
  wires:
  vecIn/1 -> Dot Product/2, Dot Product/1
  Dot Product/1 -> Sqrt/1
  Sqrt/1 -> magOut/1

== system L1_Control_with_fallback/Modified L1 Guidance - Line/Calc Nu to fly To WP A/crossproductZ ==
  vecIn2D 1 : Inport
  vecIn2D 2 : Inport  Port=2
  Demux : Demux  Outputs=2
  Demux1 : Demux  Outputs=2
  Product : Product  RndMeth=Zero
  Product1 : Product  RndMeth=Zero
  Sum2 : Sum  Inputs=|+-
  scalarOut1 : Outport
  wires:
  Product/1 -> Sum2/1
  Sum2/1 -> scalarOut1/1
  Demux1/2 -> Product/2
  Demux1/1 -> Product1/2
  vecIn2D 1/1 -> Demux/1
  Demux/2 -> Product1/1
  Demux/1 -> Product/1
  vecIn2D 2/1 -> Demux1/1
  Product1/1 -> Sum2/2

== system L1_Control_with_fallback/Modified L1 Guidance - Line/Calc Nu to fly To WP A/unitVector 2 ==
  vecIn : Inport
  Divide : Product  Inputs=*/
  Dot Product : DotProduct  InputSameDT=on  OutDataTypeStr=Inherit: Inherit via internal rule
  Sqrt : Sqrt  SaturateOnIntegerOverflow=on
  vecOut : Outport
  wires:
  vecIn/1 -> Divide/1, Dot Product/2, Dot Product/1
  Sqrt/1 -> Divide/2
  Dot Product/1 -> Sqrt/1
  Divide/1 -> vecOut/1

== system L1_Control_with_fallback/Modified L1 Guidance - Line/Calc Nu to fly To WP B/crossproductZ ==
  vecIn2D 1 : Inport
  vecIn2D 2 : Inport  Port=2
  Demux : Demux  Outputs=2
  Demux1 : Demux  Outputs=2
  Product : Product  RndMeth=Zero
  Product1 : Product  RndMeth=Zero
  Sum2 : Sum  Inputs=|+-
  scalarOut1 : Outport
  wires:
  Product1/1 -> Sum2/2
  vecIn2D 2/1 -> Demux1/1
  Demux/1 -> Product/1
  Demux/2 -> Product1/1
  vecIn2D 1/1 -> Demux/1
  Demux1/1 -> Product1/2
  Demux1/2 -> Product/2
  Sum2/1 -> scalarOut1/1
  Product/1 -> Sum2/1

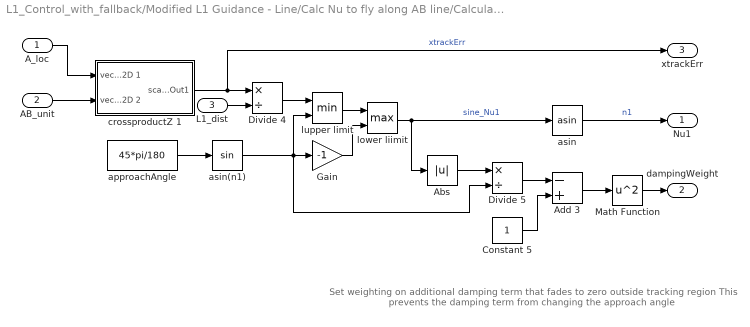
== system L1_Control_with_fallback/Modified L1 Guidance - Line/Calc Nu to fly along AB line/Calculate Nu1 Angle ==
  note: Set weighting on additional damping term that fades to zero outside tracking region
      | This prevents the damping term from changing the approach angle
  A_loc : Inport
  AB_unit : Inport  Port=2
  L1_dist : Inport  Port=3
  Abs : Abs
  Add 3 : Sum  Inputs=-+
  Constant 5 : Constant
  Divide 4 : Product  Inputs=*/
  Divide 5 : Product  Inputs=*/
  Gain : Gain  Gain=-1
  Math Function : Math  Operator=square  SaturateOnIntegerOverflow=on
  approachAngle : Constant  Value=45*pi/180
  asin : Trigonometry  Operator=asin  OutputSignalType=real
  asin(n1) : Trigonometry  OutputSignalType=real
  crossproductZ 1 : Subsystem
  lower liimit : MinMax  Function=max  Inputs=2
  lupper limit : MinMax  Inputs=2
  Nu1 : Outport
  dampingWeight : Outport  Port=2
  xtrackErr : Outport  Port=3
  wires:
  crossproductZ 1/1(scalarOut1) -> xtrackErr/1, Divide 4/1  "xtrackErr"
  approachAngle/1 -> asin(n1)/1
  Divide 4/1 -> lupper limit/1
  lupper limit/1 -> lower liimit/1
  lower liimit/1 -> Abs/1, asin/1  "sine_Nu1"
  asin(n1)/1 -> Divide 5/2, Gain/1, lupper limit/2
  Gain/1 -> lower liimit/2
  Abs/1 -> Divide 5/1
  Divide 5/1 -> Add 3/1
  Constant 5/1 -> Add 3/2
  Add 3/1 -> Math Function/1
  L1_dist/1 -> Divide 4/2
  asin/1 -> Nu1/1  "n1"
  Math Function/1 -> dampingWeight/1
  AB_unit/1 -> crossproductZ 1/2(vecIn2D 2)
  A_loc/1 -> crossproductZ 1/1(vecIn2D 1)

== system L1_Control_with_fallback/Modified L1 Guidance - Line/Calc Nu to fly along AB line/Calculate Nu2 Angle ==
  groundspeed_vector : Inport
  trackUnitVec : Inport  Port=2
  Dot Product : DotProduct  InputSameDT=on  OutDataTypeStr=Inherit: Inherit via internal rule
  Gain4 : Gain
  atan2 : Trigonometry  Operator=atan2
  crossproductZ 2 : Subsystem
  xtrackVel : Outport
  Nu2 : Outport  Port=2
  wires:
  crossproductZ 2/1(scalarOut1) -> atan2/1, Gain4/1  "xtrackVel"
  Dot Product/1 -> atan2/2  "ltrackVel"
  groundspeed_vector/1 -> crossproductZ 2/1(vecIn2D 1), Dot Product/1
  trackUnitVec/1 -> Dot Product/2, crossproductZ 2/2(vecIn2D 2)
  atan2/1 -> Nu2/1
  Gain4/1 -> xtrackVel/1

== system L1_Control_with_fallback/Modified L1 Guidance - Line/Calc Nu to fly along AB line/Calculate Nu1 Angle/crossproductZ 1 ==
  vecIn2D 1 : Inport
  vecIn2D 2 : Inport  Port=2
  Demux : Demux  Outputs=2
  Demux1 : Demux  Outputs=2
  Product : Product  RndMeth=Zero
  Product1 : Product  RndMeth=Zero
  Sum2 : Sum  Inputs=|+-
  scalarOut1 : Outport
  wires:
  Product/1 -> Sum2/1
  Sum2/1 -> scalarOut1/1
  Demux1/2 -> Product/2
  Demux1/1 -> Product1/2
  vecIn2D 1/1 -> Demux/1
  Demux/2 -> Product1/1
  Demux/1 -> Product/1
  vecIn2D 2/1 -> Demux1/1
  Product1/1 -> Sum2/2

== system L1_Control_with_fallback/Modified L1 Guidance - Line/Calc Nu to fly along AB line/Calculate Nu2 Angle/crossproductZ 2 ==
  vecIn2D 1 : Inport
  vecIn2D 2 : Inport  Port=2
  Demux : Demux  Outputs=2
  Demux1 : Demux  Outputs=2
  Product : Product  RndMeth=Zero
  Product1 : Product  RndMeth=Zero
  Sum2 : Sum  Inputs=|+-
  scalarOut1 : Outport
  wires:
  Product1/1 -> Sum2/2
  vecIn2D 2/1 -> Demux1/1
  Demux/1 -> Product/1
  Demux/2 -> Product1/1
  vecIn2D 1/1 -> Demux/1
  Demux1/1 -> Product1/2
  Demux1/2 -> Product/2
  Sum2/1 -> scalarOut1/1
  Product/1 -> Sum2/1
